simulink model "case9"  (R2024b)
settings: Solver=FixedStepAuto  StartTime=0  StopTime=1  FixedStep=1e-7  RelTol=1e-3
values from neighbouring files (symbols this model uses):
  SG_D_1_D = 0.01056    [IEEE9_case_parameters.m]    (also in case1_parameters.m; case2_parameters.m; case3_parameters.m; case4_parameters.m)
  SG_D_1_EnableSaturation = 0    [IEEE9_case_parameters.m]    (also in case1_parameters.m; case2_parameters.m; case3_parameters.m; case4_parameters.m)
  SG_D_1_f0 = 60    [IEEE9_case_parameters.m]    (also in case1_parameters.m; case2_parameters.m; case3_parameters.m; case4_parameters.m)
  SG_D_1_H = 7.5    [IEEE9_case_parameters.m]    (also in case1_parameters.m; case2_parameters.m; case3_parameters.m; case4_parameters.m)
  SG_D_1_K_A = 20    [IEEE9_case_parameters.m]    (also in case1_parameters.m; case2_parameters.m; case3_parameters.m; case4_parameters.m)
  SG_D_1_K_E = 1.000000e+1    (= 10)    [IEEE9_case_parameters.m]    (also in case1_parameters.m; case2_parameters.m; case3_parameters.m; case4_parameters.m)
  SG_D_1_K_F = 2.363    [IEEE9_case_parameters.m]    (also in case1_parameters.m; case2_parameters.m; case3_parameters.m; case4_parameters.m)
  SG_D_1_K_s = 0.5    [IEEE9_case_parameters.m]    (also in case1_parameters.m = 5; case2_parameters.m = 5; case3_parameters.m = 5; case4_parameters.m = 5)
  SG_D_1_R_a = 0.001088    [IEEE9_case_parameters.m]    (also in case1_parameters.m; case2_parameters.m; case3_parameters.m; case4_parameters.m)
  SG_D_1_S_A = 1    [IEEE9_case_parameters.m]    (also in case1_parameters.m; case2_parameters.m; case3_parameters.m; case4_parameters.m)
  SG_D_1_S_B = 0.103    [IEEE9_case_parameters.m]    (also in case1_parameters.m; case2_parameters.m; case3_parameters.m; case4_parameters.m)
  SG_D_1_S_N = 10.659857    [IEEE9_case_parameters.m]    (also in case1_parameters.m; case2_parameters.m; case3_parameters.m; case4_parameters.m)
  SG_D_1_SpeedPara = 200    [IEEE9_case_parameters.m]    (also in case1_parameters.m; case2_parameters.m; case3_parameters.m; case4_parameters.m)
  SG_D_1_T_0 = 0.720173    [IEEE9_case_parameters.m]    (also in case1_parameters.m = 0.755522; case2_parameters.m = 0.808931; case3_parameters.m = 0.869402; case4_parameters.m = 0.729316)
  SG_D_1_T_1 = 0.3    [IEEE9_case_parameters.m]    (also in case1_parameters.m; case2_parameters.m; case3_parameters.m; case4_parameters.m)
  SG_D_1_T_2 = 0.05    [IEEE9_case_parameters.m]    (also in case1_parameters.m; case2_parameters.m; case3_parameters.m; case4_parameters.m)
  SG_D_1_T_3 = 0.02    [IEEE9_case_parameters.m]    (also in case1_parameters.m; case2_parameters.m; case3_parameters.m; case4_parameters.m)
  SG_D_1_T_4 = 0.005    [IEEE9_case_parameters.m]    (also in case1_parameters.m; case2_parameters.m; case3_parameters.m; case4_parameters.m)
  SG_D_1_T_A = 0.02    [IEEE9_case_parameters.m]    (also in case1_parameters.m; case2_parameters.m; case3_parameters.m; case4_parameters.m)
  SG_D_1_T_dd = 8.000000e+0    (= 8)    [IEEE9_case_parameters.m]    (also in case1_parameters.m; case2_parameters.m; case3_parameters.m; case4_parameters.m)
  SG_D_1_T_ddd = 0.04    [IEEE9_case_parameters.m]    (also in case1_parameters.m; case2_parameters.m; case3_parameters.m; case4_parameters.m)
  SG_D_1_T_E = 0.314    [IEEE9_case_parameters.m]    (also in case1_parameters.m; case2_parameters.m; case3_parameters.m; case4_parameters.m)
  SG_D_1_T_F = 0.35    [IEEE9_case_parameters.m]    (also in case1_parameters.m; case2_parameters.m; case3_parameters.m; case4_parameters.m)
  SG_D_1_T_qd = 0.8    [IEEE9_case_parameters.m]    (also in case1_parameters.m; case2_parameters.m; case3_parameters.m; case4_parameters.m)
  SG_D_1_T_qdd = 0.02    [IEEE9_case_parameters.m]    (also in case1_parameters.m; case2_parameters.m; case3_parameters.m; case4_parameters.m)
  SG_D_1_T_speed = 0.1    [IEEE9_case_parameters.m]    (also in case1_parameters.m = 200; case2_parameters.m = 200; case3_parameters.m = 200; case4_parameters.m = 200)
  SG_D_1_T_w = 0.5    [IEEE9_case_parameters.m]    (also in case1_parameters.m; case2_parameters.m; case3_parameters.m; case4_parameters.m)
  SG_D_1_V_ref = 1.990276    [IEEE9_case_parameters.m]    (also in case1_parameters.m = 2.042296; case2_parameters.m = 2.051388; case3_parameters.m = 2.089584; case4_parameters.m = 2.01845)
  SG_D_1_w_ref = 376.991118    [IEEE9_case_parameters.m]    (also in case1_parameters.m; case2_parameters.m; case3_parameters.m; case4_parameters.m)
  SG_D_1_wb = 6.000000e+1    (= 60)    [IEEE9_case_parameters.m]    (also in case1_parameters.m; case2_parameters.m; case3_parameters.m; case4_parameters.m)
  SG_D_1_x_d = 1.9    [IEEE9_case_parameters.m]    (also in case1_parameters.m; case2_parameters.m; case3_parameters.m; case4_parameters.m)
  SG_D_1_x_dd = 0.302    [IEEE9_case_parameters.m]    (also in case1_parameters.m; case2_parameters.m; case3_parameters.m; case4_parameters.m)
  SG_D_1_x_ddd = 0.204    [IEEE9_case_parameters.m]    (also in case1_parameters.m; case2_parameters.m; case3_parameters.m; case4_parameters.m)
  SG_D_1_x_l = 0.05    [IEEE9_case_parameters.m]    (also in case1_parameters.m; case2_parameters.m; case3_parameters.m; case4_parameters.m)
  SG_D_1_x_q = 1.3    [IEEE9_case_parameters.m]    (also in case1_parameters.m; case2_parameters.m; case3_parameters.m; case4_parameters.m)
  SG_D_1_x_qd = 0.5    [IEEE9_case_parameters.m]    (also in case1_parameters.m; case2_parameters.m; case3_parameters.m; case4_parameters.m)
  SG_D_1_x_qdd = 0.3    [IEEE9_case_parameters.m]    (also in case1_parameters.m; case2_parameters.m; case3_parameters.m; case4_parameters.m)
  SG_D_2_D = 0.02    [IEEE9_case_parameters.m]    (also in case1_parameters.m; case2_parameters.m; case3_parameters.m; case4_parameters.m)
  SG_D_2_EnableSaturation = 0    [IEEE9_case_parameters.m]    (also in case1_parameters.m; case2_parameters.m; case3_parameters.m; case4_parameters.m)
  SG_D_2_f0 = 60    [IEEE9_case_parameters.m]    (also in case1_parameters.m; case2_parameters.m; case3_parameters.m; case4_parameters.m)
  SG_D_2_H = 8.000000e+0    (= 8)    [IEEE9_case_parameters.m]    (also in case1_parameters.m; case2_parameters.m; case3_parameters.m; case4_parameters.m)
  SG_D_2_K_A = 20    [IEEE9_case_parameters.m]    (also in case1_parameters.m; case2_parameters.m; case3_parameters.m; case4_parameters.m)
  SG_D_2_K_E = 1.000000e+1    (= 10)    [IEEE9_case_parameters.m]    (also in case1_parameters.m; case2_parameters.m; case3_parameters.m; case4_parameters.m)
  SG_D_2_K_F = 2.363    [IEEE9_case_parameters.m]    (also in case1_parameters.m; case2_parameters.m; case3_parameters.m; case4_parameters.m)
  SG_D_2_K_s = 0.5    [IEEE9_case_parameters.m]    (also in case1_parameters.m = 4; case2_parameters.m = 4; case3_parameters.m = 4; case4_parameters.m = 4)
  SG_D_2_R_a = 0.001088    [IEEE9_case_parameters.m]    (also in case1_parameters.m; case2_parameters.m; case3_parameters.m; case4_parameters.m)
  SG_D_2_S_A = 1    [IEEE9_case_parameters.m]    (also in case1_parameters.m; case2_parameters.m; case3_parameters.m; case4_parameters.m)
  SG_D_2_S_B = 0.103    [IEEE9_case_parameters.m]    (also in case1_parameters.m; case2_parameters.m; case3_parameters.m; case4_parameters.m)
  SG_D_2_S_N = 10.659857    [IEEE9_case_parameters.m]    (also in case1_parameters.m; case2_parameters.m; case3_parameters.m; case4_parameters.m)
  SG_D_2_SpeedPara = 200    [IEEE9_case_parameters.m]    (also in case1_parameters.m; case2_parameters.m; case3_parameters.m; case4_parameters.m)
  SG_D_2_T_0 = 1.632913    [IEEE9_case_parameters.m]    (also in case1_parameters.m = 1.632925; case2_parameters.m = 1.632915; case3_parameters.m = 1.632914; case4_parameters.m = 1.632927)
  SG_D_2_T_1 = 0.2    [IEEE9_case_parameters.m]    (also in case1_parameters.m; case2_parameters.m; case3_parameters.m; case4_parameters.m)
  SG_D_2_T_2 = 0.05    [IEEE9_case_parameters.m]    (also in case1_parameters.m; case2_parameters.m; case3_parameters.m; case4_parameters.m)
  SG_D_2_T_3 = 0.02    [IEEE9_case_parameters.m]    (also in case1_parameters.m; case2_parameters.m; case3_parameters.m; case4_parameters.m)
  SG_D_2_T_4 = 0.005    [IEEE9_case_parameters.m]    (also in case1_parameters.m; case2_parameters.m; case3_parameters.m; case4_parameters.m)
  SG_D_2_T_A = 0.02    [IEEE9_case_parameters.m]    (also in case1_parameters.m; case2_parameters.m; case3_parameters.m; case4_parameters.m)
  SG_D_2_T_dd = 7.9    [IEEE9_case_parameters.m]    (also in case1_parameters.m; case2_parameters.m; case3_parameters.m; case4_parameters.m)
  SG_D_2_T_ddd = 0.04    [IEEE9_case_parameters.m]    (also in case1_parameters.m; case2_parameters.m; case3_parameters.m; case4_parameters.m)
  SG_D_2_T_E = 0.314    [IEEE9_case_parameters.m]    (also in case1_parameters.m; case2_parameters.m; case3_parameters.m; case4_parameters.m)
  SG_D_2_T_F = 0.35    [IEEE9_case_parameters.m]    (also in case1_parameters.m; case2_parameters.m; case3_parameters.m; case4_parameters.m)
  SG_D_2_T_qd = 0.8    [IEEE9_case_parameters.m]    (also in case1_parameters.m; case2_parameters.m; case3_parameters.m; case4_parameters.m)
  SG_D_2_T_qdd = 0.015    [IEEE9_case_parameters.m]    (also in case1_parameters.m; case2_parameters.m; case3_parameters.m; case4_parameters.m)
  SG_D_2_T_speed = 0.1    [IEEE9_case_parameters.m]    (also in case1_parameters.m = 150; case2_parameters.m = 150; case3_parameters.m = 150; case4_parameters.m = 150)
  SG_D_2_T_w = 0.35    [IEEE9_case_parameters.m]    (also in case1_parameters.m; case2_parameters.m; case3_parameters.m; case4_parameters.m)
  SG_D_2_V_ref = 2.58547    [IEEE9_case_parameters.m]    (also in case1_parameters.m = 2.597896; case2_parameters.m = 2.587136; case3_parameters.m = 2.586042; case4_parameters.m = 2.599679)
  SG_D_2_w_ref = 376.991118    [IEEE9_case_parameters.m]    (also in case1_parameters.m; case2_parameters.m; case3_parameters.m; case4_parameters.m)
  SG_D_2_wb = 6.000000e+1    (= 60)    [IEEE9_case_parameters.m]    (also in case1_parameters.m; case2_parameters.m; case3_parameters.m; case4_parameters.m)
  SG_D_2_x_d = 1.8    [IEEE9_case_parameters.m]    (also in case1_parameters.m; case2_parameters.m; case3_parameters.m; case4_parameters.m)
  SG_D_2_x_dd = 0.302    [IEEE9_case_parameters.m]    (also in case1_parameters.m; case2_parameters.m; case3_parameters.m; case4_parameters.m)
  SG_D_2_x_ddd = 0.204    [IEEE9_case_parameters.m]    (also in case1_parameters.m; case2_parameters.m; case3_parameters.m; case4_parameters.m)
  SG_D_2_x_l = 0.05    [IEEE9_case_parameters.m]    (also in case1_parameters.m; case2_parameters.m; case3_parameters.m; case4_parameters.m)
  SG_D_2_x_q = 1.25    [IEEE9_case_parameters.m]    (also in case1_parameters.m; case2_parameters.m; case3_parameters.m; case4_parameters.m)
  SG_D_2_x_qd = 0.5    [IEEE9_case_parameters.m]    (also in case1_parameters.m; case2_parameters.m; case3_parameters.m; case4_parameters.m)
  SG_D_2_x_qdd = 0.3    [IEEE9_case_parameters.m]    (also in case1_parameters.m; case2_parameters.m; case3_parameters.m; case4_parameters.m)
  SG_D_3_D = 0.02    [IEEE9_case_parameters.m]    (also in case1_parameters.m; case2_parameters.m; case3_parameters.m; case4_parameters.m)
  SG_D_3_EnableSaturation = 0    [IEEE9_case_parameters.m]    (also in case1_parameters.m; case2_parameters.m; case3_parameters.m; case4_parameters.m)
  SG_D_3_f0 = 60    [IEEE9_case_parameters.m]    (also in case1_parameters.m; case2_parameters.m; case3_parameters.m; case4_parameters.m)
  SG_D_3_H = 7.7    [IEEE9_case_parameters.m]    (also in case1_parameters.m; case2_parameters.m; case3_parameters.m; case4_parameters.m)
  SG_D_3_K_A = 20    [IEEE9_case_parameters.m]    (also in case1_parameters.m; case2_parameters.m; case3_parameters.m; case4_parameters.m)
  SG_D_3_K_E = 1.000000e+1    (= 10)    [IEEE9_case_parameters.m]    (also in case1_parameters.m; case2_parameters.m; case3_parameters.m; case4_parameters.m)
  SG_D_3_K_F = 2.363    [IEEE9_case_parameters.m]    (also in case1_parameters.m; case2_parameters.m; case3_parameters.m; case4_parameters.m)
  SG_D_3_K_s = 0.2    [IEEE9_case_parameters.m]    (also in case1_parameters.m = 2; case2_parameters.m = 2; case3_parameters.m = 2; case4_parameters.m = 2)
  SG_D_3_R_a = 0.001088    [IEEE9_case_parameters.m]    (also in case1_parameters.m; case2_parameters.m; case3_parameters.m; case4_parameters.m)
  SG_D_3_S_A = 1    [IEEE9_case_parameters.m]    (also in case1_parameters.m; case2_parameters.m; case3_parameters.m; case4_parameters.m)
  SG_D_3_S_B = 0.103    [IEEE9_case_parameters.m]    (also in case1_parameters.m; case2_parameters.m; case3_parameters.m; case4_parameters.m)
  SG_D_3_S_N = 10.659857    [IEEE9_case_parameters.m]    (also in case1_parameters.m; case2_parameters.m; case3_parameters.m; case4_parameters.m)
  SG_D_3_SpeedPara = 200    [IEEE9_case_parameters.m]    (also in case1_parameters.m; case2_parameters.m; case3_parameters.m; case4_parameters.m)
  SG_D_3_T_0 = 0.850788    [IEEE9_case_parameters.m]    (also in case1_parameters.m = 0.850786; case2_parameters.m = 0.850787; case3_parameters.m; case4_parameters.m = 0.850786)
  SG_D_3_T_1 = 0.2    [IEEE9_case_parameters.m]    (also in case1_parameters.m; case2_parameters.m; case3_parameters.m; case4_parameters.m)
  SG_D_3_T_2 = 0.05    [IEEE9_case_parameters.m]    (also in case1_parameters.m; case2_parameters.m; case3_parameters.m; case4_parameters.m)
  SG_D_3_T_3 = 0.02    [IEEE9_case_parameters.m]    (also in case1_parameters.m; case2_parameters.m; case3_parameters.m; case4_parameters.m)
  SG_D_3_T_4 = 0.005    [IEEE9_case_parameters.m]    (also in case1_parameters.m; case2_parameters.m; case3_parameters.m; case4_parameters.m)
  SG_D_3_T_A = 0.02    [IEEE9_case_parameters.m]    (also in case1_parameters.m; case2_parameters.m; case3_parameters.m; case4_parameters.m)
  SG_D_3_T_dd = 8.1    [IEEE9_case_parameters.m]    (also in case1_parameters.m; case2_parameters.m; case3_parameters.m; case4_parameters.m)
  SG_D_3_T_ddd = 0.04    [IEEE9_case_parameters.m]    (also in case1_parameters.m; case2_parameters.m; case3_parameters.m; case4_parameters.m)
  SG_D_3_T_E = 0.314    [IEEE9_case_parameters.m]    (also in case1_parameters.m; case2_parameters.m; case3_parameters.m; case4_parameters.m)
  SG_D_3_T_F = 0.35    [IEEE9_case_parameters.m]    (also in case1_parameters.m; case2_parameters.m; case3_parameters.m; case4_parameters.m)
  SG_D_3_T_qd = 0.8    [IEEE9_case_parameters.m]    (also in case1_parameters.m; case2_parameters.m; case3_parameters.m; case4_parameters.m)
  SG_D_3_T_qdd = 0.015    [IEEE9_case_parameters.m]    (also in case1_parameters.m; case2_parameters.m; case3_parameters.m; case4_parameters.m)
  SG_D_3_T_speed = 0.1    [IEEE9_case_parameters.m]    (also in case1_parameters.m = 180; case2_parameters.m = 180; case3_parameters.m = 180; case4_parameters.m = 180)
  SG_D_3_T_w = 0.4    [IEEE9_case_parameters.m]    (also in case1_parameters.m; case2_parameters.m; case3_parameters.m; case4_parameters.m)
  SG_D_3_V_ref = 1.892727    [IEEE9_case_parameters.m]    (also in case1_parameters.m = 1.906439; case2_parameters.m = 1.895535; case3_parameters.m = 1.892105; case4_parameters.m = 1.906598)
  SG_D_3_w_ref = 376.991118    [IEEE9_case_parameters.m]    (also in case1_parameters.m; case2_parameters.m; case3_parameters.m; case4_parameters.m)
  SG_D_3_wb = 6.000000e+1    (= 60)    [IEEE9_case_parameters.m]    (also in case1_parameters.m; case2_parameters.m; case3_parameters.m; case4_parameters.m)
  SG_D_3_x_d = 1.85    [IEEE9_case_parameters.m]    (also in case1_parameters.m; case2_parameters.m; case3_parameters.m; case4_parameters.m)
  SG_D_3_x_dd = 0.302    [IEEE9_case_parameters.m]    (also in case1_parameters.m; case2_parameters.m; case3_parameters.m; case4_parameters.m)
  SG_D_3_x_ddd = 0.204    [IEEE9_case_parameters.m]    (also in case1_parameters.m; case2_parameters.m; case3_parameters.m; case4_parameters.m)
  SG_D_3_x_l = 0.05    [IEEE9_case_parameters.m]    (also in case1_parameters.m; case2_parameters.m; case3_parameters.m; case4_parameters.m)
  SG_D_3_x_q = 1.2    [IEEE9_case_parameters.m]    (also in case1_parameters.m; case2_parameters.m; case3_parameters.m; case4_parameters.m)
  SG_D_3_x_qd = 0.5    [IEEE9_case_parameters.m]    (also in case1_parameters.m; case2_parameters.m; case3_parameters.m; case4_parameters.m)
  SG_D_3_x_qdd = 0.3    [IEEE9_case_parameters.m]    (also in case1_parameters.m; case2_parameters.m; case3_parameters.m; case4_parameters.m)
(part 1 of 12)
settings Model: Creator=Greg  LastModifiedBy=Greg

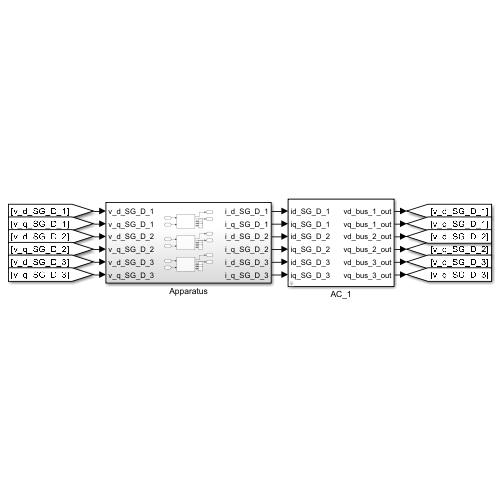
[thumbnail: Simulink's stored preview of the top-level diagram]
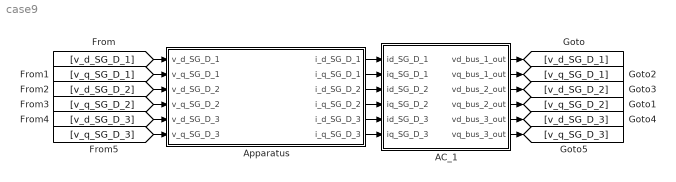
== system case9 ==
  AC_1 : Subsystem  mask(AC_1){}
      mask help: Parameters Interface of AC_1
  Apparatus : Subsystem
  wires:
  Apparatus/1(i_d_SG_D_1) -> AC_1/1(id_SG_D_1)
  Apparatus/2(i_q_SG_D_1) -> AC_1/2(iq_SG_D_1)
  Apparatus/3(i_d_SG_D_2) -> AC_1/3(id_SG_D_2)
  Apparatus/4(i_q_SG_D_2) -> AC_1/4(iq_SG_D_2)
  Apparatus/5(i_d_SG_D_3) -> AC_1/5(id_SG_D_3)
  Apparatus/6(i_q_SG_D_3) -> AC_1/6(iq_SG_D_3)
  AC_1/1(vd_bus_1_out) -> [v_d_SG_D_1]
  [v_d_SG_D_1] -> Apparatus/1(v_d_SG_D_1)
  AC_1/4(vq_bus_2_out) -> [v_q_SG_D_2]
  AC_1/6(vq_bus_3_out) -> [v_q_SG_D_3]
  AC_1/5(vd_bus_3_out) -> [v_d_SG_D_3]
  AC_1/3(vd_bus_2_out) -> [v_d_SG_D_2]
  AC_1/2(vq_bus_1_out) -> [v_q_SG_D_1]
  [v_q_SG_D_1] -> Apparatus/2(v_q_SG_D_1)
  [v_d_SG_D_2] -> Apparatus/3(v_d_SG_D_2)
  [v_q_SG_D_2] -> Apparatus/4(v_q_SG_D_2)
  [v_d_SG_D_3] -> Apparatus/5(v_d_SG_D_3)
  [v_q_SG_D_3] -> Apparatus/6(v_q_SG_D_3)

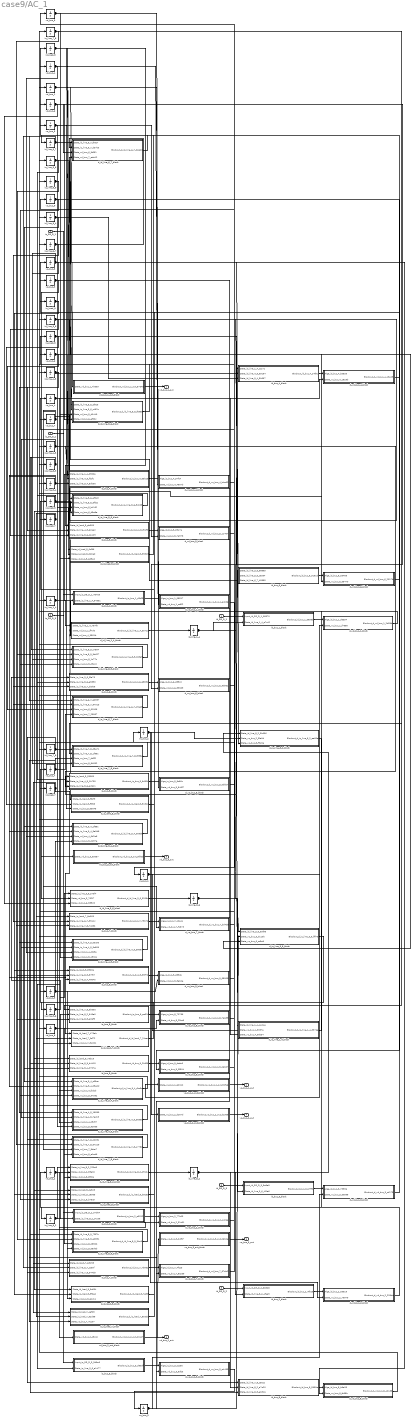
== system case9/AC_1 ==
  id_SG_D_1 : Inport
  iq_SG_D_1 : Inport  Port=2
  id_SG_D_2 : Inport  Port=3
  iq_SG_D_2 : Inport  Port=4
  id_SG_D_3 : Inport  Port=5
  iq_SG_D_3 : Inport  Port=6
  d_id_line_1_4_block : Subsystem
  d_id_line_3_6_block : Subsystem
  d_id_line_4_5_block : Subsystem
  d_id_line_5_6_block : Subsystem
  d_id_line_6_7_block : Subsystem
  d_id_line_7_8_block : Subsystem
  d_id_line_8_2_block : Subsystem
  d_id_line_8_9_block : Subsystem
  d_id_line_9_4_block : Subsystem
  d_id_load_5_block : Subsystem
  d_id_load_7_block : Subsystem
  d_id_load_9_block : Subsystem
  d_iq_line_1_4_block : Subsystem
  d_iq_line_3_6_block : Subsystem
  d_iq_line_4_5_block : Subsystem
  d_iq_line_5_6_block : Subsystem
  d_iq_line_6_7_block : Subsystem
  d_iq_line_7_8_block : Subsystem
  d_iq_line_8_2_block : Subsystem
  d_iq_line_8_9_block : Subsystem
  d_iq_line_9_4_block : Subsystem
  d_iq_load_5_block : Subsystem
  d_iq_load_7_block : Subsystem
  d_iq_load_9_block : Subsystem
  d_vd_bus_1_block : Subsystem
  d_vd_bus_2_block : Subsystem
  d_vd_bus_3_block : Subsystem
  d_vd_bus_4_block : Subsystem
  d_vd_bus_5_block : Subsystem
  d_vd_bus_6_block : Subsystem
  d_vd_bus_7_block : Subsystem
  d_vd_bus_8_block : Subsystem
  d_vd_bus_9_block : Subsystem
  d_vq_bus_1_block : Subsystem
  d_vq_bus_2_block : Subsystem
  d_vq_bus_3_block : Subsystem
  d_vq_bus_4_block : Subsystem
  d_vq_bus_5_block : Subsystem
  d_vq_bus_6_block : Subsystem
  d_vq_bus_7_block : Subsystem
  d_vq_bus_8_block : Subsystem
  d_vq_bus_9_block : Subsystem
  id_bus_1_block : Subsystem
  id_bus_2_block : Subsystem
  id_bus_3_block : Subsystem
  id_bus_4_block : Subsystem
  id_bus_5_block : Subsystem
  id_bus_6_block : Subsystem
  id_bus_7_block : Subsystem
  id_bus_8_block : Subsystem
  id_bus_9_block : Subsystem
  id_line_1_4 : Integrator  InitialCondition=0.8773
  id_line_3_6 : Integrator  InitialCondition=0.8449
  id_line_4_5 : Integrator  InitialCondition=0.3786
  id_line_5_6 : Integrator  InitialCondition=-0.5815
  id_line_6_7 : Integrator  InitialCondition=0.2671
  id_line_7_8 : Integrator  InitialCondition=-0.7938
  id_line_8_2 : Integrator  InitialCondition=-1.6302
  id_line_8_9 : Integrator  InitialCondition=0.8467
  id_line_9_4 : Integrator  InitialCondition=-0.4901
  id_load_5 : Integrator  InitialCondition=0.9381806603503355
  id_load_7 : Integrator  InitialCondition=1.05880148787843
  id_load_9 : Integrator  InitialCondition=1.3150449069818613
  iq_bus_1_block : Subsystem
  iq_bus_2_block : Subsystem
  iq_bus_3_block : Subsystem
  iq_bus_4_block : Subsystem
  iq_bus_5_block : Subsystem
  iq_bus_6_block : Subsystem
  iq_bus_7_block : Subsystem
  iq_bus_8_block : Subsystem
  iq_bus_9_block : Subsystem
  iq_line_1_4 : Integrator  InitialCondition=-0.2207
  iq_line_3_6 : Integrator  InitialCondition=0.1073
  iq_line_4_5 : Integrator  InitialCondition=-0.0777
  iq_line_5_6 : Integrator  InitialCondition=0.0412
  iq_line_6_7 : Integrator  InitialCondition=-0.1362
  iq_line_7_8 : Integrator  InitialCondition=0.0312
  iq_line_8_2 : Integrator  InitialCondition=-0.1209
  iq_line_8_9 : Integrator  InitialCondition=-0.0747
  iq_line_9_4 : Integrator  InitialCondition=0.3078
  iq_load_5 : Integrator  InitialCondition=-0.3699474910908063
  iq_load_7 : Integrator  InitialCondition=-0.34407273505131625
  iq_load_9 : Integrator  InitialCondition=-0.6127437202587428
  vd_bus_1 : Integrator  InitialCondition=1.0
  vd_bus_1_out_block : Subsystem
  vd_bus_2 : Integrator  InitialCondition=0.9888568778126388
  vd_bus_2_out_block : Subsystem
  vd_bus_3 : Integrator  InitialCondition=0.9979745831484245
  vd_bus_3_out_block : Subsystem
  vd_bus_4 : Integrator  InitialCondition=0.9871040048196629
  vd_bus_5 : Integrator  InitialCondition=0.9729598653196824
  vd_bus_6 : Integrator  InitialCondition=1.0043528995717355
  vd_bus_7 : Integrator  InitialCondition=0.9870181241657715
  vd_bus_8 : Integrator  InitialCondition=0.9965197929948038
  vd_bus_9 : Integrator  InitialCondition=0.9553110095191761
  vq_bus_1 : Integrator  InitialCondition=0.0
  vq_bus_1_out_block : Subsystem
  vq_bus_2 : Integrator  InitialCondition=0.1488693225706359
  vq_bus_2_out_block : Subsystem
  vq_bus_3 : Integrator  InitialCondition=0.06361392449557196
  vq_bus_3_out_block : Subsystem
  vq_bus_4 : Integrator  InitialCondition=-0.05126585087833766
  vq_bus_5 : Integrator  InitialCondition=-0.08519092525017519
  vq_bus_6 : Integrator  InitialCondition=0.013384513311058882
  vq_bus_7 : Integrator  InitialCondition=-0.012199182448088602
  vq_bus_8 : Integrator  InitialCondition=0.04550367844668248
  vq_bus_9 : Integrator  InitialCondition=-0.09023381410544636
  vd_bus_1_out : Outport
  vq_bus_1_out : Outport  Port=2
  vd_bus_2_out : Outport  Port=3
  vq_bus_2_out : Outport  Port=4
  vd_bus_3_out : Outport  Port=5
  vq_bus_3_out : Outport  Port=6
  wires:
  iq_line_9_4/1 -> d_id_line_9_4_block/2(State_iq_line_9_4_5e3d8), d_iq_line_9_4_block/2(State_iq_line_9_4_05e2d), iq_bus_4_block/3(State_iq_line_9_4_5dba6), iq_bus_9_block/3(State_iq_line_9_4_4804a)
  vq_bus_6/1 -> d_iq_line_3_6_block/3(State_vq_bus_6_cc5e9), d_iq_line_5_6_block/4(State_vq_bus_6_d5e8e), d_iq_line_6_7_block/3(State_vq_bus_6_61006), d_vd_bus_6_block/2(State_vq_bus_6_65470)
  d_id_line_1_4_block/1(Blockout_d_id_line_1_4_3a712) -> id_line_1_4/1
  vq_bus_2_out_block/1(Blockout_vq_bus_2_out_d1306) -> vq_bus_2_out/1
  iq_SG_D_3/1 -> iq_bus_3_block/1(Input_iq_SG_D_3_3d9a6)
  id_bus_1_block/1(Blockout_id_bus_1_e658d) -> d_vd_bus_1_block/1(Alge_id_bus_1_d6354)
  vd_bus_6/1 -> d_id_line_5_6_block/4(State_vd_bus_6_efdbc), d_id_line_3_6_block/3(State_vd_bus_6_98520), d_id_line_6_7_block/3(State_vd_bus_6_9df61), d_vq_bus_6_block/2(State_vd_bus_6_933d9)
  iq_bus_2_block/1(Blockout_iq_bus_2_a9312) -> d_vq_bus_2_block/1(Alge_iq_bus_2_77b03)
  d_vq_bus_3_block/1(Blockout_d_vq_bus_3_a4433) -> vq_bus_3/1
  iq_line_3_6/1 -> iq_bus_3_block/2(State_iq_line_3_6_e1477), iq_bus_6_block/1(State_iq_line_3_6_f0e75), d_id_line_3_6_block/1(State_iq_line_3_6_a7af4)
  id_SG_D_2/1 -> id_bus_2_block/1(Input_id_SG_D_2_88308)
  iq_load_9/1 -> d_iq_load_9_block/2(State_iq_load_9_18565), iq_bus_9_block/1(State_iq_load_9_8900a), d_id_load_9_block/2(State_iq_load_9_9f0e2)
  d_vd_bus_4_block/1(Blockout_d_vd_bus_4_13a25) -> vd_bus_4/1
  id_SG_D_3/1 -> id_bus_3_block/1(Input_id_SG_D_3_5e5e9)
  d_iq_line_8_2_block/1(Blockout_d_iq_line_8_2_ea60e) -> iq_line_8_2/1
  vd_bus_3_out_block/1(Blockout_vd_bus_3_out_0fd0d) -> vd_bus_3_out/1
  iq_line_6_7/1 -> d_id_line_6_7_block/2(State_iq_line_6_7_d37ba), d_iq_line_6_7_block/2(State_iq_line_6_7_97013), iq_bus_7_block/2(State_iq_line_6_7_3541c), iq_bus_6_block/3(State_iq_line_6_7_dc0b6)
  iq_SG_D_2/1 -> iq_bus_2_block/1(Input_iq_SG_D_2_07d64)
  id_SG_D_1/1 -> id_bus_1_block/1(Input_id_SG_D_1_08570)
  id_bus_9_block/1(Blockout_id_bus_9_2b9f8) -> d_vd_bus_9_block/1(Alge_id_bus_9_dcda6)
  iq_SG_D_1/1 -> iq_bus_1_block/1(Input_iq_SG_D_1_4e7e5)
  d_id_line_3_6_block/1(Blockout_d_id_line_3_6_9206c) -> id_line_3_6/1
  iq_bus_9_block/1(Blockout_iq_bus_9_35f70) -> d_vq_bus_9_block/1(Alge_iq_bus_9_d89c6)
  d_vq_bus_7_block/1(Blockout_d_vq_bus_7_bd4da) -> vq_bus_7/1
  id_line_5_6/1 -> id_bus_6_block/2(State_id_line_5_6_ca554), d_iq_line_5_6_block/1(State_id_line_5_6_afd48), d_id_line_5_6_block/1(State_id_line_5_6_cf92e), id_bus_5_block/3(State_id_line_5_6_da129)
  id_bus_7_block/1(Blockout_id_bus_7_7b061) -> d_vd_bus_7_block/1(Alge_id_bus_7_4fc23)
  d_vq_bus_5_block/1(Blockout_d_vq_bus_5_0bbb7) -> vq_bus_5/1
  vq_bus_3_out_block/1(Blockout_vq_bus_3_out_26b2e) -> vq_bus_3_out/1
  iq_bus_8_block/1(Blockout_iq_bus_8_ea31f) -> d_vq_bus_8_block/1(Alge_iq_bus_8_70786)
  id_bus_3_block/1(Blockout_id_bus_3_b7ff3) -> d_vd_bus_3_block/1(Alge_id_bus_3_75936)
  id_bus_8_block/1(Blockout_id_bus_8_5999e) -> d_vd_bus_8_block/1(Alge_id_bus_8_b8a05)
  d_id_line_5_6_block/1(Blockout_d_id_line_5_6_fe5e5) -> id_line_5_6/1
  d_iq_load_5_block/1(Blockout_d_iq_load_5_51512) -> iq_load_5/1
  d_vd_bus_6_block/1(Blockout_d_vd_bus_6_2017b) -> vd_bus_6/1
  iq_line_8_9/1 -> d_id_line_8_9_block/2(State_iq_line_8_9_a0851), d_iq_line_8_9_block/2(State_iq_line_8_9_9dd27), iq_bus_9_block/2(State_iq_line_8_9_87f07), iq_bus_8_block/3(State_iq_line_8_9_a06f9)
  vd_bus_1/1 -> d_vq_bus_1_block/2(State_vd_bus_1_cc6f2), d_id_line_1_4_block/2(State_vd_bus_1_ff7d0), vd_bus_1_out_block/1(State_vd_bus_1_7b6a9)
  vq_bus_9/1 -> d_iq_line_8_9_block/4(State_vq_bus_9_c542c), d_iq_line_9_4_block/4(State_vq_bus_9_57552), d_vd_bus_9_block/2(State_vq_bus_9_f0504), d_iq_load_9_block/3(State_vq_bus_9_b75c9)
  iq_bus_7_block/1(Blockout_iq_bus_7_79b7d) -> d_vq_bus_7_block/1(Alge_iq_bus_7_10ac4)
  iq_bus_5_block/1(Blockout_iq_bus_5_6d5f4) -> d_vq_bus_5_block/1(Alge_iq_bus_5_8c66c)
  id_load_5/1 -> d_id_load_5_block/1(State_id_load_5_0cf96), d_iq_load_5_block/1(State_id_load_5_f81f9), id_bus_5_block/1(State_id_load_5_eb383)
  iq_bus_3_block/1(Blockout_iq_bus_3_d80df) -> d_vq_bus_3_block/1(Alge_iq_bus_3_cc23e)
  d_id_load_7_block/1(Blockout_d_id_load_7_24cac) -> id_load_7/1
  iq_bus_6_block/1(Blockout_iq_bus_6_68831) -> d_vq_bus_6_block/1(Alge_iq_bus_6_d852c)
  vq_bus_3/1 -> d_vd_bus_3_block/2(State_vq_bus_3_e0598), vq_bus_3_out_block/1(State_vq_bus_3_04fbf), d_iq_line_3_6_block/2(State_vq_bus_3_d110b)
  vq_bus_1_out_block/1(Blockout_vq_bus_1_out_92f46) -> vq_bus_1_out/1
  vd_bus_1_out_block/1(Blockout_vd_bus_1_out_57e40) -> vd_bus_1_out/1
  id_bus_4_block/1(Blockout_id_bus_4_24f5c) -> d_vd_bus_4_block/1(Alge_id_bus_4_ba533)
  id_line_4_5/1 -> id_bus_4_block/2(State_id_line_4_5_e9164), d_id_line_4_5_block/1(State_id_line_4_5_0ac06), d_iq_line_4_5_block/1(State_id_line_4_5_16899), id_bus_5_block/2(State_id_line_4_5_62aa2)
  id_bus_6_block/1(Blockout_id_bus_6_9161d) -> d_vd_bus_6_block/1(Alge_id_bus_6_03468)
  id_bus_5_block/1(Blockout_id_bus_5_f01f3) -> d_vd_bus_5_block/1(Alge_id_bus_5_0947a)
  iq_line_7_8/1 -> d_iq_line_7_8_block/2(State_iq_line_7_8_1f96c), iq_bus_7_block/3(State_iq_line_7_8_7cd8b), d_id_line_7_8_block/2(State_iq_line_7_8_67229), iq_bus_8_block/1(State_iq_line_7_8_eb6ae)
  id_line_6_7/1 -> d_id_line_6_7_block/1(State_id_line_6_7_fa0c7), d_iq_line_6_7_block/1(State_id_line_6_7_6b997), id_bus_6_block/3(State_id_line_6_7_45885), id_bus_7_block/2(State_id_line_6_7_cc3af)
  id_bus_2_block/1(Blockout_id_bus_2_4fbc8) -> d_vd_bus_2_block/1(Alge_id_bus_2_03e19)
  iq_bus_4_block/1(Blockout_iq_bus_4_63b2e) -> d_vq_bus_4_block/1(Alge_iq_bus_4_57fc4)
  iq_bus_1_block/1(Blockout_iq_bus_1_d5df9) -> d_vq_bus_1_block/1(Alge_iq_bus_1_08517)
  vd_bus_4/1 -> d_vq_bus_4_block/2(State_vd_bus_4_4807b), d_id_line_1_4_block/3(State_vd_bus_4_3581b), d_id_line_4_5_block/3(State_vd_bus_4_c0c9a), d_id_line_9_4_block/3(State_vd_bus_4_6d2a8)
  vd_bus_2_out_block/1(Blockout_vd_bus_2_out_204c7) -> vd_bus_2_out/1
  d_iq_load_9_block/1(Blockout_d_iq_load_9_b92e3) -> iq_load_9/1
  vd_bus_8/1 -> d_vq_bus_8_block/2(State_vd_bus_8_2f4e8), d_id_line_7_8_block/4(State_vd_bus_8_e1ed6), d_id_line_8_9_block/3(State_vd_bus_8_2850b), d_id_line_8_2_block/3(State_vd_bus_8_8fc0a)
  id_line_9_4/1 -> id_bus_4_block/3(State_id_line_9_4_5b567), d_id_line_9_4_block/1(State_id_line_9_4_2f88c), d_iq_line_9_4_block/1(State_id_line_9_4_c69ca), id_bus_9_block/3(State_id_line_9_4_0707e)
  vq_bus_8/1 -> d_iq_line_8_2_block/3(State_vq_bus_8_f943e), d_iq_line_8_9_block/3(State_vq_bus_8_1c77b), d_vd_bus_8_block/2(State_vq_bus_8_fa58b), d_iq_line_7_8_block/4(State_vq_bus_8_84832)
  d_iq_line_8_9_block/1(Blockout_d_iq_line_8_9_3c3a9) -> iq_line_8_9/1
  iq_line_4_5/1 -> d_id_line_4_5_block/2(State_iq_line_4_5_5c689), iq_bus_4_block/2(State_iq_line_4_5_fdcfc), iq_bus_5_block/2(State_iq_line_4_5_1b735), d_iq_line_4_5_block/2(State_iq_line_4_5_7ec19)
  d_vd_bus_9_block/1(Blockout_d_vd_bus_9_26b07) -> vd_bus_9/1
  vq_bus_7/1 -> d_vd_bus_7_block/2(State_vq_bus_7_8c2e9), d_iq_line_6_7_block/4(State_vq_bus_7_29567), d_iq_line_7_8_block/3(State_vq_bus_7_ddff2), d_iq_load_7_block/3(State_vq_bus_7_4c107)
  d_id_line_8_2_block/1(Blockout_d_id_line_8_2_d9124) -> id_line_8_2/1
  d_iq_line_5_6_block/1(Blockout_d_iq_line_5_6_5c2d3) -> iq_line_5_6/1
  d_vq_bus_1_block/1(Blockout_d_vq_bus_1_ac2d6) -> vq_bus_1/1
  id_line_8_9/1 -> id_bus_8_block/3(State_id_line_8_9_eb516), d_id_line_8_9_block/1(State_id_line_8_9_7f57b), id_bus_9_block/2(State_id_line_8_9_b4415), d_iq_line_8_9_block/1(State_id_line_8_9_c7584)
  id_line_8_2/1 -> d_iq_line_8_2_block/1(State_id_line_8_2_3b696), id_bus_2_block/2(State_id_line_8_2_4faa5), id_bus_8_block/2(State_id_line_8_2_a7a20)
  iq_line_8_2/1 -> d_id_line_8_2_block/1(State_iq_line_8_2_220e3), iq_bus_2_block/2(State_iq_line_8_2_c72a6), iq_bus_8_block/2(State_iq_line_8_2_645e0)
  id_line_7_8/1 -> id_bus_8_block/1(State_id_line_7_8_c3e2c), d_id_line_7_8_block/1(State_id_line_7_8_2009c), d_iq_line_7_8_block/1(State_id_line_7_8_d8e71), id_bus_7_block/3(State_id_line_7_8_e44d5)
  vq_bus_1/1 -> d_vd_bus_1_block/2(State_vq_bus_1_f7898), vq_bus_1_out_block/1(State_vq_bus_1_621b2), d_iq_line_1_4_block/2(State_vq_bus_1_3337a)
  vd_bus_9/1 -> d_id_load_9_block/3(State_vd_bus_9_61c11), d_id_line_8_9_block/4(State_vd_bus_9_05d0b), d_id_line_9_4_block/4(State_vd_bus_9_2d37e), d_vq_bus_9_block/2(State_vd_bus_9_9eb2e)
  id_load_9/1 -> d_id_load_9_block/1(State_id_load_9_9c654), d_iq_load_9_block/1(State_id_load_9_ca328), id_bus_9_block/1(State_id_load_9_75b19)
  id_line_3_6/1 -> d_iq_line_3_6_block/1(State_id_line_3_6_aaf98), id_bus_3_block/2(State_id_line_3_6_41fe6), id_bus_6_block/1(State_id_line_3_6_98865)
  iq_line_5_6/1 -> d_id_line_5_6_block/2(State_iq_line_5_6_c462c), d_iq_line_5_6_block/2(State_iq_line_5_6_efdcc), iq_bus_5_block/3(State_iq_line_5_6_ad611), iq_bus_6_block/2(State_iq_line_5_6_e5890)
  id_line_1_4/1 -> d_iq_line_1_4_block/1(State_id_line_1_4_4a24e), id_bus_1_block/2(State_id_line_1_4_a7c42), id_bus_4_block/1(State_id_line_1_4_cc172)
  iq_line_1_4/1 -> d_id_line_1_4_block/1(State_iq_line_1_4_797f0), iq_bus_1_block/2(State_iq_line_1_4_643e1), iq_bus_4_block/1(State_iq_line_1_4_0500a)
  iq_load_7/1 -> d_id_load_7_block/2(State_iq_load_7_faf72), d_iq_load_7_block/2(State_iq_load_7_52d58), iq_bus_7_block/1(State_iq_load_7_bb003)
  id_load_7/1 -> d_id_load_7_block/1(State_id_load_7_475ab), d_iq_load_7_block/1(State_id_load_7_4efb5), id_bus_7_block/1(State_id_load_7_63198)
  iq_load_5/1 -> d_id_load_5_block/2(State_iq_load_5_0d2e0), d_iq_load_5_block/2(State_iq_load_5_ffc98), iq_bus_5_block/1(State_iq_load_5_53083)
  vd_bus_3/1 -> vd_bus_3_out_block/1(State_vd_bus_3_a5a57), d_id_line_3_6_block/2(State_vd_bus_3_76f17), d_vq_bus_3_block/2(State_vd_bus_3_6cfca)
  vd_bus_7/1 -> d_vq_bus_7_block/2(State_vd_bus_7_f1873), d_id_load_7_block/3(State_vd_bus_7_54001), d_id_line_6_7_block/4(State_vd_bus_7_ede12), d_id_line_7_8_block/3(State_vd_bus_7_8dca7)
  vd_bus_2/1 -> d_vq_bus_2_block/2(State_vd_bus_2_31c31), vd_bus_2_out_block/1(State_vd_bus_2_c52cc), d_id_line_8_2_block/2(State_vd_bus_2_59e3c)
  vd_bus_5/1 -> d_vq_bus_5_block/2(State_vd_bus_5_846f7), d_id_load_5_block/3(State_vd_bus_5_6d5a2), d_id_line_4_5_block/4(State_vd_bus_5_153c4), d_id_line_5_6_block/3(State_vd_bus_5_d0449)
  d_id_line_9_4_block/1(Blockout_d_id_line_9_4_009d8) -> id_line_9_4/1
  vq_bus_5/1 -> d_vd_bus_5_block/2(State_vq_bus_5_7a578), d_iq_load_5_block/3(State_vq_bus_5_63e45), d_iq_line_4_5_block/4(State_vq_bus_5_9266e), d_iq_line_5_6_block/3(State_vq_bus_5_b416f)
  vq_bus_4/1 -> d_vd_bus_4_block/2(State_vq_bus_4_1829b), d_iq_line_1_4_block/3(State_vq_bus_4_a6b34), d_iq_line_4_5_block/3(State_vq_bus_4_25c97), d_iq_line_9_4_block/3(State_vq_bus_4_f2dcb)
  vq_bus_2/1 -> d_vd_bus_2_block/2(State_vq_bus_2_79979), d_iq_line_8_2_block/2(State_vq_bus_2_3fe0d), vq_bus_2_out_block/1(State_vq_bus_2_d267d)
  d_id_load_5_block/1(Blockout_d_id_load_5_39313) -> id_load_5/1
  d_id_load_9_block/1(Blockout_d_id_load_9_7efdf) -> id_load_9/1
  d_id_line_4_5_block/1(Blockout_d_id_line_4_5_38067) -> id_line_4_5/1
  d_id_line_6_7_block/1(Blockout_d_id_line_6_7_b6620) -> id_line_6_7/1
  d_iq_line_1_4_block/1(Blockout_d_iq_line_1_4_3376e) -> iq_line_1_4/1
  d_iq_line_6_7_block/1(Blockout_d_iq_line_6_7_15ad5) -> iq_line_6_7/1
  d_iq_line_9_4_block/1(Blockout_d_iq_line_9_4_dbc5a) -> iq_line_9_4/1
  d_id_line_7_8_block/1(Blockout_d_id_line_7_8_47780) -> id_line_7_8/1
  d_id_line_8_9_block/1(Blockout_d_id_line_8_9_34a3f) -> id_line_8_9/1
  d_vq_bus_6_block/1(Blockout_d_vq_bus_6_9d5e1) -> vq_bus_6/1
  d_iq_line_3_6_block/1(Blockout_d_iq_line_3_6_fff78) -> iq_line_3_6/1
  d_iq_line_4_5_block/1(Blockout_d_iq_line_4_5_383ee) -> iq_line_4_5/1
  d_iq_line_7_8_block/1(Blockout_d_iq_line_7_8_fd98e) -> iq_line_7_8/1
  d_iq_load_7_block/1(Blockout_d_iq_load_7_8aad1) -> iq_load_7/1
  d_vd_bus_1_block/1(Blockout_d_vd_bus_1_2d89b) -> vd_bus_1/1
  d_vd_bus_2_block/1(Blockout_d_vd_bus_2_239dc) -> vd_bus_2/1
  d_vd_bus_3_block/1(Blockout_d_vd_bus_3_cd175) -> vd_bus_3/1
  d_vd_bus_5_block/1(Blockout_d_vd_bus_5_11407) -> vd_bus_5/1
  d_vd_bus_7_block/1(Blockout_d_vd_bus_7_67ab2) -> vd_bus_7/1
  d_vd_bus_8_block/1(Blockout_d_vd_bus_8_4b188) -> vd_bus_8/1
  d_vq_bus_2_block/1(Blockout_d_vq_bus_2_4c26a) -> vq_bus_2/1
  d_vq_bus_4_block/1(Blockout_d_vq_bus_4_b4e62) -> vq_bus_4/1
  d_vq_bus_8_block/1(Blockout_d_vq_bus_8_7a639) -> vq_bus_8/1
  d_vq_bus_9_block/1(Blockout_d_vq_bus_9_68009) -> vq_bus_9/1

== system case9/Apparatus ==
  v_d_SG_D_1 : Inport
  v_q_SG_D_1 : Inport  Port=2
  v_d_SG_D_2 : Inport  Port=3
  v_q_SG_D_2 : Inport  Port=4
  v_d_SG_D_3 : Inport  Port=5
  v_q_SG_D_3 : Inport  Port=6
  SG_D_1 : Subsystem  mask(SG_D_1){T_0=SG_D_1_T_0, w_ref=SG_D_1_w_ref, V_ref=SG_D_1_V_ref, x_d=SG_D_1_x_d, x_dd=SG_D_1_x_dd, x_ddd=SG_D_1_x_ddd, x_q=SG_D_1_x_q, x_qd=SG_D_1_x_qd, x_qdd=SG_D_1_x_qdd, x_l=SG_D_1_x_l, R_a=SG_D_1_R_a, T_dd=SG_D_1_T_dd, T_ddd=SG_D_1_T_ddd, T_qd=SG_D_1_T_qd, T_qdd=SG_D_1_T_qdd, H=SG_D_1_H, D=SG_D_1_D, SpeedPara=SG_D_1_SpeedPara, K_A=SG_D_1_K_A, EnableSaturation=SG_D_1_EnableSaturation, f0=SG_D_1_f0, T_speed=SG_D_1_T_speed, T_E=SG_D_1_T_E, T_A=SG_D_1_T_A, T_F=SG_D_1_T_F, K_E=SG_D_1_K_E, K_F=SG_D_1_K_F, K_s=SG_D_1_K_s, T_1=SG_D_1_T_1, T_2=SG_D_1_T_2, T_3=SG_D_1_T_3, T_4=SG_D_1_T_4, T_w=SG_D_1_T_w, wb=SG_D_1_wb, S_A=SG_D_1_S_A, S_B=SG_D_1_S_B, S_N=SG_D_1_S_N}
      mask help: Parameters Interface of SG_D_1
  SG_D_2 : Subsystem  mask(SG_D_2){T_0=SG_D_2_T_0, w_ref=SG_D_2_w_ref, V_ref=SG_D_2_V_ref, x_d=SG_D_2_x_d, x_dd=SG_D_2_x_dd, x_ddd=SG_D_2_x_ddd, x_q=SG_D_2_x_q, x_qd=SG_D_2_x_qd, x_qdd=SG_D_2_x_qdd, x_l=SG_D_2_x_l, R_a=SG_D_2_R_a, T_dd=SG_D_2_T_dd, T_ddd=SG_D_2_T_ddd, T_qd=SG_D_2_T_qd, T_qdd=SG_D_2_T_qdd, H=SG_D_2_H, D=SG_D_2_D, SpeedPara=SG_D_2_SpeedPara, K_A=SG_D_2_K_A, EnableSaturation=SG_D_2_EnableSaturation, f0=SG_D_2_f0, T_speed=SG_D_2_T_speed, T_E=SG_D_2_T_E, T_A=SG_D_2_T_A, T_F=SG_D_2_T_F, K_E=SG_D_2_K_E, K_F=SG_D_2_K_F, K_s=SG_D_2_K_s, T_1=SG_D_2_T_1, T_2=SG_D_2_T_2, T_3=SG_D_2_T_3, T_4=SG_D_2_T_4, T_w=SG_D_2_T_w, wb=SG_D_2_wb, S_A=SG_D_2_S_A, S_B=SG_D_2_S_B, S_N=SG_D_2_S_N}
      mask help: Parameters Interface of SG_D_2
  SG_D_3 : Subsystem  mask(SG_D_3){T_0=SG_D_3_T_0, w_ref=SG_D_3_w_ref, V_ref=SG_D_3_V_ref, x_d=SG_D_3_x_d, x_dd=SG_D_3_x_dd, x_ddd=SG_D_3_x_ddd, x_q=SG_D_3_x_q, x_qd=SG_D_3_x_qd, x_qdd=SG_D_3_x_qdd, x_l=SG_D_3_x_l, R_a=SG_D_3_R_a, T_dd=SG_D_3_T_dd, T_ddd=SG_D_3_T_ddd, T_qd=SG_D_3_T_qd, T_qdd=SG_D_3_T_qdd, H=SG_D_3_H, D=SG_D_3_D, SpeedPara=SG_D_3_SpeedPara, K_A=SG_D_3_K_A, EnableSaturation=SG_D_3_EnableSaturation, f0=SG_D_3_f0, T_speed=SG_D_3_T_speed, T_E=SG_D_3_T_E, T_A=SG_D_3_T_A, T_F=SG_D_3_T_F, K_E=SG_D_3_K_E, K_F=SG_D_3_K_F, K_s=SG_D_3_K_s, T_1=SG_D_3_T_1, T_2=SG_D_3_T_2, T_3=SG_D_3_T_3, T_4=SG_D_3_T_4, T_w=SG_D_3_T_w, wb=SG_D_3_wb, S_A=SG_D_3_S_A, S_B=SG_D_3_S_B, S_N=SG_D_3_S_N}
      mask help: Parameters Interface of SG_D_3
  Terminator{,1..8} (9 alike) : Terminator
  i_d_SG_D_1 : Outport
  i_q_SG_D_1 : Outport  Port=2
  i_d_SG_D_2 : Outport  Port=3
  i_q_SG_D_2 : Outport  Port=4
  i_d_SG_D_3 : Outport  Port=5
  i_q_SG_D_3 : Outport  Port=6
  wires:
  SG_D_2/2(i_q_SG_D_2) -> i_q_SG_D_2/1
  SG_D_1/1(i_d_SG_D_1) -> i_d_SG_D_1/1
  v_d_SG_D_1/1 -> SG_D_1/1(v_d_SG_D_1)
  SG_D_2/1(i_d_SG_D_2) -> i_d_SG_D_2/1
  SG_D_3/2(i_q_SG_D_3) -> i_q_SG_D_3/1
  SG_D_3/1(i_d_SG_D_3) -> i_d_SG_D_3/1
  SG_D_1/2(i_q_SG_D_1) -> i_q_SG_D_1/1
  v_q_SG_D_3/1 -> SG_D_3/2(v_q_SG_D_3)
  v_d_SG_D_2/1 -> SG_D_2/1(v_d_SG_D_2)
  v_q_SG_D_1/1 -> SG_D_1/2(v_q_SG_D_1)
  v_q_SG_D_2/1 -> SG_D_2/2(v_q_SG_D_2)
  v_d_SG_D_3/1 -> SG_D_3/1(v_d_SG_D_3)
  SG_D_1/3(T_e_SG_D_1) -> Terminator/1
  SG_D_1/4(w_SG_D_1_out) -> Terminator1/1
  SG_D_1/5(theta_SG_D_1_out) -> Terminator2/1
  SG_D_2/3(T_e_SG_D_2) -> Terminator3/1
  SG_D_2/4(w_SG_D_2_out) -> Terminator4/1
  SG_D_2/5(theta_SG_D_2_out) -> Terminator5/1
  SG_D_3/3(T_e_SG_D_3) -> Terminator6/1
  SG_D_3/4(w_SG_D_3_out) -> Terminator7/1
  SG_D_3/5(theta_SG_D_3_out) -> Terminator8/1

== system case9/AC_1/d_id_line_1_4_block ==
  note: d_id_line_1_4 in case9
      | $376.991118430775\,\mathrm{iq}_{\mathrm{line},1,4}+6451.28815726045\,\mathrm{vd}_{\mathrm{bus},1}-6451.28815726045\,\mathrm{vd}_{\mathrm{bus},4}$
      | Automatically generated on 2025-10-31 19:35:40 .
  State_iq_line_1_4_797f0 : Inport
  State_vd_bus_1_ff7d0 : Inport  Port=2
  State_vd_bus_4_3581b : Inport  Port=3
  Add_1c15f : Sum
  Constant_376.991118430775_c2257 : Constant  Value=376.991118430775
  Constant_6451.28815726045_0a8e7 : Constant  Value=6451.28815726045
  Constant_6451.28815726045_0ddfa : Constant  Value=6451.28815726045
  Product_32285 : Product
  Product_a25f3 : Product
  Product_cd978 : Product
  Subtract_4a07f : Sum  Inputs=+-
  Blockout_d_id_line_1_4_3a712 : Outport
  wires:
  Constant_376.991118430775_c2257/1 -> Product_cd978/1
  Product_32285/1 -> Add_1c15f/2
  State_iq_line_1_4_797f0/1 -> Product_cd978/2
  Subtract_4a07f/1 -> Blockout_d_id_line_1_4_3a712/1
  Constant_6451.28815726045_0a8e7/1 -> Product_32285/1
  Product_cd978/1 -> Add_1c15f/1
  State_vd_bus_1_ff7d0/1 -> Product_32285/2
  Constant_6451.28815726045_0ddfa/1 -> Product_a25f3/1
  State_vd_bus_4_3581b/1 -> Product_a25f3/2
  Add_1c15f/1 -> Subtract_4a07f/1
  Product_a25f3/1 -> Subtract_4a07f/2

== system case9/AC_1/d_id_line_3_6_block ==
  note: d_id_line_3_6 in case9
      | $376.991118430775\,\mathrm{iq}_{\mathrm{line},3,6}+6341.19791566897\,\mathrm{vd}_{\mathrm{bus},3}-6341.19791566897\,\mathrm{vd}_{\mathrm{bus},6}$
      | Automatically generated on 2025-10-31 19:35:42 .
  State_iq_line_3_6_a7af4 : Inport
  State_vd_bus_3_76f17 : Inport  Port=2
  State_vd_bus_6_98520 : Inport  Port=3
  Add_a36cd : Sum
  Constant_376.991118430775_a01cc : Constant  Value=376.991118430775
  Constant_6341.19791566897_4e785 : Constant  Value=6341.19791566897
  Constant_6341.19791566897_ee108 : Constant  Value=6341.19791566897
  Product_41c3b : Product
  Product_ae2ef : Product
  Product_d543d : Product
  Subtract_466b8 : Sum  Inputs=+-
  Blockout_d_id_line_3_6_9206c : Outport
  wires:
  State_vd_bus_3_76f17/1 -> Product_41c3b/2
  Constant_376.991118430775_a01cc/1 -> Product_d543d/1
  Product_41c3b/1 -> Add_a36cd/2
  State_iq_line_3_6_a7af4/1 -> Product_d543d/2
  Constant_6341.19791566897_4e785/1 -> Product_41c3b/1
  Product_d543d/1 -> Add_a36cd/1
  Constant_6341.19791566897_ee108/1 -> Product_ae2ef/1
  State_vd_bus_6_98520/1 -> Product_ae2ef/2
  Add_a36cd/1 -> Subtract_466b8/1
  Product_ae2ef/1 -> Subtract_466b8/2
  Subtract_466b8/1 -> Blockout_d_id_line_3_6_9206c/1

== system case9/AC_1/d_id_line_4_5_block ==
  note: d_id_line_4_5 in case9
      | $376.991118430775\,\mathrm{iq}_{\mathrm{line},4,5}-73.5192666060942\,\mathrm{id}_{\mathrm{line},4,5}+4039.06736802393\,\mathrm{vd}_{\mathrm{bus},4}-4039.06736802393\,\mathrm{vd}_{\mathrm{bus},5}$
      | Automatically generated on 2025-10-31 19:35:41 .
  State_id_line_4_5_0ac06 : Inport
  State_iq_line_4_5_5c689 : Inport  Port=2
  State_vd_bus_4_c0c9a : Inport  Port=3
  State_vd_bus_5_153c4 : Inport  Port=4
  Add_695ee : Sum
  Add_b9d3f : Sum
  Constant_-73.5192666060942_2d289 : Constant  Value=-73.5192666060942
  Constant_376.991118430775_8116c : Constant  Value=376.991118430775
  Constant_4039.06736802393_f0698 : Constant  Value=4039.06736802393
  Constant_4039.06736802393_f5fdf : Constant  Value=4039.06736802393
  Product_0d4c9 : Product
  Product_13625 : Product
  Product_38b6d : Product
  Product_75658 : Product
  Subtract_132c0 : Sum  Inputs=+-
  Blockout_d_id_line_4_5_38067 : Outport
  wires:
  Constant_-73.5192666060942_2d289/1 -> Product_13625/1
  Product_0d4c9/1 -> Add_695ee/2
  State_id_line_4_5_0ac06/1 -> Product_13625/2
  Constant_376.991118430775_8116c/1 -> Product_0d4c9/1
  State_iq_line_4_5_5c689/1 -> Product_0d4c9/2
  Product_13625/1 -> Add_695ee/1
  Constant_4039.06736802393_f0698/1 -> Product_75658/1
  State_vd_bus_4_c0c9a/1 -> Product_75658/2
  Add_695ee/1 -> Add_b9d3f/1
  Product_75658/1 -> Add_b9d3f/2
  Constant_4039.06736802393_f5fdf/1 -> Product_38b6d/1
  State_vd_bus_5_153c4/1 -> Product_38b6d/2
  Add_b9d3f/1 -> Subtract_132c0/1
  Product_38b6d/1 -> Subtract_132c0/2
  Subtract_132c0/1 -> Blockout_d_id_line_4_5_38067/1

== system case9/AC_1/d_id_line_5_6_block ==
  note: d_id_line_5_6 in case9
      | $376.991118430775\,\mathrm{iq}_{\mathrm{line},5,6}-91.2758230389848\,\mathrm{id}_{\mathrm{line},5,6}+2185.8482226953\,\mathrm{vd}_{\mathrm{bus},5}-2185.8482226953\,\mathrm{vd}_{\mathrm{bus},6}$
      | Automatically generated on 2025-10-31 19:35:42 .
  State_id_line_5_6_cf92e : Inport
  State_iq_line_5_6_c462c : Inport  Port=2
  State_vd_bus_5_d0449 : Inport  Port=3
  State_vd_bus_6_efdbc : Inport  Port=4
  Add_356cd : Sum
  Add_8f1cb : Sum
  Constant_-91.2758230389848_81505 : Constant  Value=-91.2758230389848
  Constant_2185.8482226953_4547a : Constant  Value=2185.8482226953
  Constant_2185.8482226953_7c2ab : Constant  Value=2185.8482226953
  Constant_376.991118430775_4d139 : Constant  Value=376.991118430775
  Product_8f138 : Product
  Product_a7480 : Product
  Product_d679a : Product
  Product_db793 : Product
  Subtract_5faa0 : Sum  Inputs=+-
  Blockout_d_id_line_5_6_fe5e5 : Outport
  wires:
  Constant_-91.2758230389848_81505/1 -> Product_a7480/1
  Product_d679a/1 -> Add_356cd/2
  State_id_line_5_6_cf92e/1 -> Product_a7480/2
  Constant_376.991118430775_4d139/1 -> Product_d679a/1
  Product_a7480/1 -> Add_356cd/1
  State_iq_line_5_6_c462c/1 -> Product_d679a/2
  Constant_2185.8482226953_7c2ab/1 -> Product_8f138/1
  Product_db793/1 -> Subtract_5faa0/2
  State_vd_bus_5_d0449/1 -> Product_8f138/2
  Add_356cd/1 -> Add_8f1cb/1
  Product_8f138/1 -> Add_8f1cb/2
  Constant_2185.8482226953_4547a/1 -> Product_db793/1
  State_vd_bus_6_efdbc/1 -> Product_db793/2
  Add_8f1cb/1 -> Subtract_5faa0/1
  Subtract_5faa0/1 -> Blockout_d_id_line_5_6_fe5e5/1

== system case9/AC_1/d_id_line_6_7_block ==
  note: d_id_line_6_7 in case9
      | $376.991118430775\,\mathrm{iq}_{\mathrm{line},6,7}-46.9706425538935\,\mathrm{id}_{\mathrm{line},6,7}+3686.4503755774\,\mathrm{vd}_{\mathrm{bus},6}-3686.4503755774\,\mathrm{vd}_{\mathrm{bus},7}$
      | Automatically generated on 2025-10-31 19:35:43 .
  State_id_line_6_7_fa0c7 : Inport
  State_iq_line_6_7_d37ba : Inport  Port=2
  State_vd_bus_6_9df61 : Inport  Port=3
  State_vd_bus_7_ede12 : Inport  Port=4
  Add_0182f : Sum
  Add_99eae : Sum
  Constant_-46.9706425538935_97953 : Constant  Value=-46.9706425538935
  Constant_3686.4503755774_09060 : Constant  Value=3686.4503755774
  Constant_3686.4503755774_58e62 : Constant  Value=3686.4503755774
  Constant_376.991118430775_2df46 : Constant  Value=376.991118430775
  Product_7716f : Product
  Product_bd52f : Product
  Product_fa866 : Product
  Product_ff410 : Product
  Subtract_6e985 : Sum  Inputs=+-
  Blockout_d_id_line_6_7_b6620 : Outport
  wires:
  Constant_-46.9706425538935_97953/1 -> Product_ff410/1
  Product_7716f/1 -> Add_99eae/2
  State_id_line_6_7_fa0c7/1 -> Product_ff410/2
  Constant_376.991118430775_2df46/1 -> Product_7716f/1
  State_iq_line_6_7_d37ba/1 -> Product_7716f/2
  Product_ff410/1 -> Add_99eae/1
  Constant_3686.4503755774_58e62/1 -> Product_fa866/1
  State_vd_bus_6_9df61/1 -> Product_fa866/2
  Add_99eae/1 -> Add_0182f/1
  Product_fa866/1 -> Add_0182f/2
  Constant_3686.4503755774_09060/1 -> Product_bd52f/1
  State_vd_bus_7_ede12/1 -> Product_bd52f/2
  Add_0182f/1 -> Subtract_6e985/1
  Product_bd52f/1 -> Subtract_6e985/2
  Subtract_6e985/1 -> Blockout_d_id_line_6_7_b6620/1

== system case9/AC_1/d_id_line_7_8_block ==
  note: d_id_line_7_8 in case9
      | $376.991118430775\,\mathrm{iq}_{\mathrm{line},7,8}-46.9706425538935\,\mathrm{id}_{\mathrm{line},7,8}+5161.03052580836\,\mathrm{vd}_{\mathrm{bus},7}-5161.03052580836\,\mathrm{vd}_{\mathrm{bus},8}$
      | Automatically generated on 2025-10-31 19:35:44 .
  State_id_line_7_8_2009c : Inport
  State_iq_line_7_8_67229 : Inport  Port=2
  State_vd_bus_7_8dca7 : Inport  Port=3
  State_vd_bus_8_e1ed6 : Inport  Port=4
  Add_7b634 : Sum
  Add_d7225 : Sum
  Constant_-46.9706425538935_09ed1 : Constant  Value=-46.9706425538935
  Constant_376.991118430775_25d2c : Constant  Value=376.991118430775
  Constant_5161.03052580836_2e632 : Constant  Value=5161.03052580836
  Constant_5161.03052580836_45bb4 : Constant  Value=5161.03052580836
  Product_65fa1 : Product
  Product_6c08f : Product
  Product_7b510 : Product
  Product_8ccd9 : Product
  Subtract_a6668 : Sum  Inputs=+-
  Blockout_d_id_line_7_8_47780 : Outport
  wires:
  Constant_-46.9706425538935_09ed1/1 -> Product_8ccd9/1
  Product_6c08f/1 -> Add_d7225/2
  State_id_line_7_8_2009c/1 -> Product_8ccd9/2
  Constant_376.991118430775_25d2c/1 -> Product_6c08f/1
  Product_8ccd9/1 -> Add_d7225/1
  State_iq_line_7_8_67229/1 -> Product_6c08f/2
  Constant_5161.03052580836_2e632/1 -> Product_65fa1/1
  State_vd_bus_7_8dca7/1 -> Product_65fa1/2
  Add_d7225/1 -> Add_7b634/1
  Product_65fa1/1 -> Add_7b634/2
  Constant_5161.03052580836_45bb4/1 -> Product_7b510/1
  State_vd_bus_8_e1ed6/1 -> Product_7b510/2
  Add_7b634/1 -> Subtract_a6668/1
  Product_7b510/1 -> Subtract_a6668/2
  Subtract_a6668/1 -> Blockout_d_id_line_7_8_47780/1

== system case9/AC_1/d_id_line_8_2_block ==
  note: d_id_line_8_2 in case9
      | $376.991118430775\,\mathrm{iq}_{\mathrm{line},8,2}-5945.50716573123\,\mathrm{vd}_{\mathrm{bus},2}+5945.50716573123\,\mathrm{vd}_{\mathrm{bus},8}$
      | Automatically generated on 2025-10-31 19:35:45 .
  State_iq_line_8_2_220e3 : Inport
  State_vd_bus_2_59e3c : Inport  Port=2
  State_vd_bus_8_8fc0a : Inport  Port=3
  Add_ae313 : Sum
  Constant_376.991118430775_cff1f : Constant  Value=376.991118430775
  Constant_5945.50716573123_19739 : Constant  Value=5945.50716573123
  Constant_5945.50716573123_da0a8 : Constant  Value=5945.50716573123
  Product_bb867 : Product
  Product_c0a0d : Product
  Product_ee5c0 : Product
  Subtract_0eebd : Sum  Inputs=+-
  Blockout_d_id_line_8_2_d9124 : Outport
  wires:
  State_vd_bus_2_59e3c/1 -> Product_c0a0d/2
  Constant_376.991118430775_cff1f/1 -> Product_ee5c0/1
  Product_c0a0d/1 -> Subtract_0eebd/2
  State_iq_line_8_2_220e3/1 -> Product_ee5c0/2
  Constant_5945.50716573123_da0a8/1 -> Product_c0a0d/1
  Product_ee5c0/1 -> Subtract_0eebd/1
  Constant_5945.50716573123_19739/1 -> Product_bb867/1
  State_vd_bus_8_8fc0a/1 -> Product_bb867/2
  Subtract_0eebd/1 -> Add_ae313/1
  Product_bb867/1 -> Add_ae313/2
  Add_ae313/1 -> Blockout_d_id_line_8_2_d9124/1
